simulink model "UserInputs"  (R2017b)
settings: Solver=FixedStepDiscrete  StartTime=0.0  StopTime=10.0  FixedStep=0.08  RelTol=1e-3
libraries: MATLAB_Function_lib x1
settings Model: Creator=hbourbou  LastModifiedBy=hbourbou

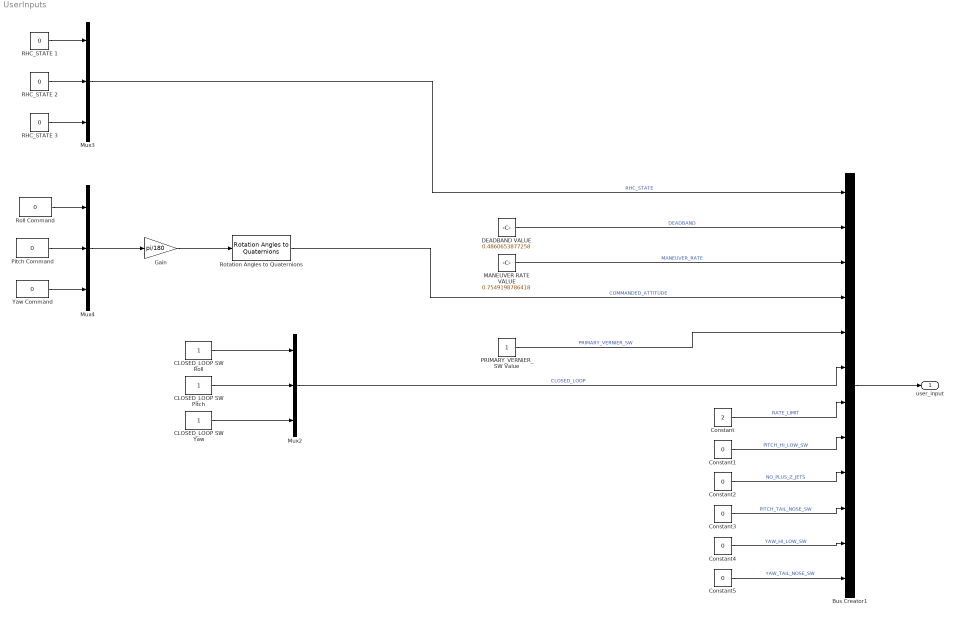
== system UserInputs ==
  Bus Creator1 : BusCreator  Inputs=12  OutDataTypeStr=Bus: user_inputsBus  NonVirtualBus=on
  CLOSED_LOOP SW Pitch : Constant  OutDataTypeStr=boolean
  CLOSED_LOOP SW Roll : Constant  OutDataTypeStr=boolean
  CLOSED_LOOP SW Yaw : Constant  OutDataTypeStr=boolean
  Constant : Constant  Value=2
  Constant{1..5} (5 alike) : Constant  Value=0  OutDataTypeStr=boolean
  DEADBAND VALUE : Constant  Value=0.4860653877258
  Gain : Gain  Gain=pi/180
  MANEUVER RATE VALUE : Constant  Value=0.7549198786418
  Mux2 : Mux  Inputs=3
  Mux3 : Mux  Inputs=3
  Mux4 : Mux  Inputs=3
  PRIMARY_VERNIER_SW Value : Constant  OutDataTypeStr=boolean
  Pitch Command : Constant  Value=0
  RHC_STATE 1 : Constant  Value=0  OutDataTypeStr=int8
  RHC_STATE 2 : Constant  Value=0  OutDataTypeStr=int8
  RHC_STATE 3 : Constant  Value=0  OutDataTypeStr=int8
  Roll Command : Constant  Value=0
  Rotation Angles to Quaternions : MATLAB_Function_lib/Rotation Angles to Quaternions
  Yaw Command : Constant  Value=0
  user_input : Outport  OutDataTypeStr=Bus: user_inputsBus
  wires:
  CLOSED_LOOP SW Yaw/1 -> Mux2/3
  RHC_STATE 2/1 -> Mux3/2
  Yaw Command/1 -> Mux4/3
  CLOSED_LOOP SW Pitch/1 -> Mux2/2
  PRIMARY_VERNIER_SW Value/1 -> Bus Creator1/5  "PRIMARY_VERNIER_SW"
  Constant1/1 -> Bus Creator1/8  "PITCH_HI_LOW_SW"
  Pitch Command/1 -> Mux4/2
  Mux2/1 -> Bus Creator1/6  "CLOSED_LOOP"
  RHC_STATE 3/1 -> Mux3/3
  Rotation Angles to Quaternions/1 -> Bus Creator1/4  "COMMANDED_ATTITUDE"
  Constant3/1 -> Bus Creator1/10  "PITCH_TAIL_NOSE_SW"
  Gain/1 -> Rotation Angles to Quaternions/1
  Constant5/1 -> Bus Creator1/12  "YAW_TAIL_NOSE_SW"
  MANEUVER RATE VALUE/1 -> Bus Creator1/3  "MANEUVER_RATE"
  CLOSED_LOOP SW Roll/1 -> Mux2/1
  Constant4/1 -> Bus Creator1/11  "YAW_HI_LOW_SW"
  Mux3/1 -> Bus Creator1/1  "RHC_STATE"
  Roll Command/1 -> Mux4/1
  DEADBAND VALUE/1 -> Bus Creator1/2  "DEADBAND"
  Mux4/1 -> Gain/1
  RHC_STATE 1/1 -> Mux3/1
  Constant/1 -> Bus Creator1/7  "RATE_LIMIT"
  Constant2/1 -> Bus Creator1/9  "NO_PLUS_Z_JETS"
  Bus Creator1/1 -> user_input/1
